simulink model "modified"  (R2017b)
settings: Solver=VariableStepAuto  StartTime=0.0  StopTime=1600  FixedStep=0.1  RelTol=1e-3
InitFcn:
  | A=[0 1;5 -6];
  | b=[4;4];
  | C=[2 3];
  | U=ctrb(A,b);
  | rank(U);
  | Ad=[0 1;-256 -32];
  | H=[1 0];
  | U2=obsv(Ad,H);
  | rank(U2);
  | 
  | M=sylv(A,-Ad,b*H);
  | K=H*inv(M)
  | 
  | k0g=0.02;
  | k1g=1;
  | k2g=3;
  | k3g=5;
  | A0g=[0 1 0 0;
  |           0 0 1 0;
  |           0 0 0 1;
  |         -k0g -k1g -k2g -k3g ];
  | b0g=[0;0;0;1];
  | Am=A-b*K
settings Model: Creator=lida  LastModifiedBy=lida

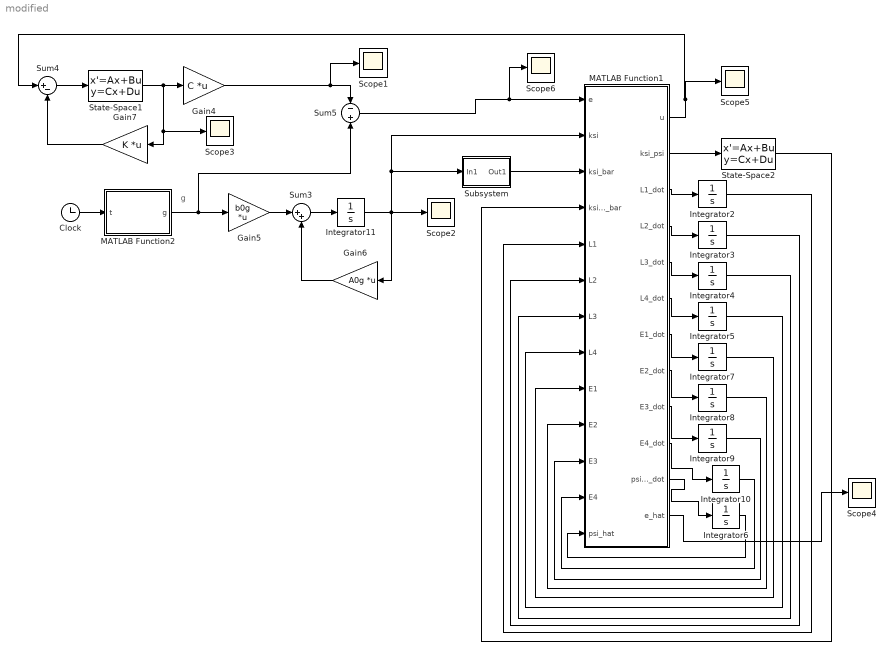
== system modified ==
  note: g
  Clock : Clock
  Gain4 : Gain  Gain=C  Multiplication=Matrix(K*u)
  Gain5 : Gain  Gain=b0g  Multiplication=Matrix(K*u)
  Gain6 : Gain  Gain=A0g  Multiplication=Matrix(K*u)
  Gain7 : Gain  Gain=K  Multiplication=Matrix(K*u)
  Integrator{7..10} (4 alike) : Integrator
  Integrator{2..6,11} (6 alike) : Integrator  InitialCondition=zeros(4,1)
  MATLAB Function1 : MATLAB Function  TreatAsAtomicUnit=on
  MATLAB Function2 : MATLAB Function  TreatAsAtomicUnit=on
  Scope{1..6} (6 alike) : Scope
  State-Space1 : StateSpace  A=A  B=b  C=eye(2)  D=[0;0]  InitialCondition=[1;0]
  State-Space2 : StateSpace  A=Am  B=b  C=C  D=0  InitialCondition=0
  Subsystem : Subsystem
  Sum3 : Sum  Inputs=|++
  Sum4 : Sum  Inputs=|+-
  Sum5 : Sum  Inputs=-+
  wires:
  Sum5/1 -> Scope6/1, MATLAB Function1/1(e)
  MATLAB Function1/1(u) -> Scope5/1, Sum4/1
  MATLAB Function1/3(L1_dot) -> Integrator2/1
  MATLAB Function1/4(L2_dot) -> Integrator3/1
  MATLAB Function1/5(L3_dot) -> Integrator4/1
  MATLAB Function1/6(L4_dot) -> Integrator5/1
  Integrator2/1 -> MATLAB Function1/5(L1)
  Integrator3/1 -> MATLAB Function1/6(L2)
  Integrator4/1 -> MATLAB Function1/7(L3)
  Integrator5/1 -> MATLAB Function1/8(L4)
  MATLAB Function1/7(E1_dot) -> Integrator7/1
  MATLAB Function1/8(E2_dot) -> Integrator8/1
  MATLAB Function1/9(E3_dot) -> Integrator9/1
  MATLAB Function1/10(E4_dot) -> Integrator10/1
  Integrator10/1 -> MATLAB Function1/12(E4)
  Integrator9/1 -> MATLAB Function1/11(E3)
  Integrator8/1 -> MATLAB Function1/10(E2)
  Integrator7/1 -> MATLAB Function1/9(E1)
  Sum3/1 -> Integrator11/1
  Subsystem/1(Out1) -> MATLAB Function1/3(ksi_bar)
  Gain6/1 -> Sum3/2
  MATLAB Function2/1(g) -> Sum5/2, Gain5/1
  Sum4/1 -> State-Space1/1
  Gain7/1 -> Sum4/2
  State-Space1/1 -> Scope3/1, Gain7/1, Gain4/1
  Gain5/1 -> Sum3/1
  Clock/1 -> MATLAB Function2/1(t)
  MATLAB Function1/11(psi_hat_dot) -> Integrator6/1
  Integrator6/1 -> MATLAB Function1/13(psi_hat)
  MATLAB Function1/2(ksi_psi) -> State-Space2/1
  State-Space2/1 -> MATLAB Function1/4(ksi_psi_bar)
  Gain4/1 -> Scope1/1, Sum5/1
  Integrator11/1 -> Gain6/1, Scope2/1, MATLAB Function1/2(ksi), Subsystem/1(In1)
  MATLAB Function1/12(e_hat) -> Scope4/1

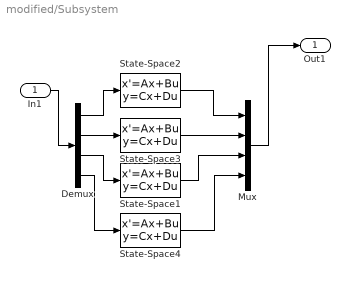
== system modified/Subsystem ==
  In1 : Inport
  Demux : Demux
  Mux : Mux
  State-Space{1..4} (4 alike) : StateSpace  A=Am  B=b  C=C  D=0  InitialCondition=0
  Out1 : Outport
  wires:
  In1/1 -> Demux/1
  Demux/1 -> State-Space2/1
  Mux/1 -> Out1/1
  State-Space2/1 -> Mux/1
  State-Space3/1 -> Mux/2
  Demux/2 -> State-Space3/1
  Demux/3 -> State-Space1/1
  Demux/4 -> State-Space4/1
  State-Space1/1 -> Mux/3
  State-Space4/1 -> Mux/4

== matlab function modified/MATLAB Function1 ==
  data: u output; ksi_psi output; L1_dot output; L2_dot output; L3_dot output; L4_dot output; E1_dot output; E2_dot output; E3_dot output; E4_dot output; e input; ksi input; ksi_bar input; ksi_psi_bar input; L1 input; L2 input; L3 input; L4 input; E1 input; E2 input; E3 input; E4 input; psi_hat input; psi_hat_dot output; e_hat output
function [u,ksi_psi,L1_dot,L2_dot,L3_dot,L4_dot,E1_dot,E2_dot,E3_dot,E4_dot,psi_hat_dot,e_hat] = fcn(e,ksi,ksi_bar,ksi_psi_bar,L1,L2,L3,L4,E1,E2,E3,E4,psi_hat)
gamma0=10000;gamma=0.001;mu1=1;mu2=2;mu3=3;mu4=4;
% y_hat=theta_hat'*omega;
% theta_tilda=theta-theta_hat;
% e_y=y-y_hat;
ksi_psi=ksi'*psi_hat;
% psi_dot=gamma*ksi_bar*e_hat;

L1_dot=-mu1*L1+ksi;
L2_dot=-mu2*L2+ksi;
L3_dot=-mu3*L3+ksi;
L4_dot=-mu4*L4+ksi;
L=[L1';L2';L3';L4'];
Le=L'*L;

E1_dot=-mu1*E1+e+psi_hat'*ksi;
E2_dot=-mu2*E2+e+psi_hat'*ksi;
E3_dot=-mu3*E3+e+psi_hat'*ksi;
E4_dot=-mu1*E4+e+psi_hat'*ksi;
E=[E1;E2;E3;E4];

% x_hat=x_bar*psi_hat;

e_hat=e-psi_hat'*ksi_bar+ksi_psi_bar;
psi_hat_dot=gamma0*ksi*e_hat+gamma*L'*(E-L*psi_hat);

u=psi_hat'*ksi;

== matlab function modified/MATLAB Function2 ==
  data: t input; g output
function g = fcn(t)

g=5*sin(3*t-2)*sin(6*t+10);
